simulink library "Vehicule"  (R2018a)
settings: Solver=VariableStepAuto  StartTime=0.0  StopTime=10.0  RelTol=1e-3
values from neighbouring files (symbols this model uses):
  cycleLife = (0:1:500)    [ImportationRoute.m]
  dod = interp1(temperature, deepOfDischarge, temp)    [ImportationRoute.m]
  dod2 = interp1(cyLi, dischargeCapacity, cycleLife)    [ImportationRoute.m]
  temp = (-20:1:40)    [ImportationRoute.m]
libraries: $bdroot x3, simulink x2
settings Model: Creator=thomas.moser  LastModifiedBy=thomas.moser

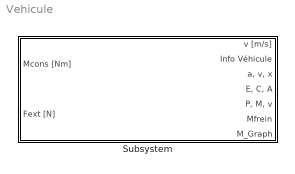
== system Vehicule ==
  Subsystem : Subsystem  mask{m=2250, mp=80, rr=0.33, s=1, cx=0.5, crr=0.015, mlimit=660, alimit=3, Vmin=25/3.6, Vmax=250/3.6, r=9.73, nr=0.9, nm=0.89, Pmax=310380, Mmax=660, nc=0.89, cb=98, soc=100, tempExt=25, nbrCycle=0}
      mask prompts: m "Poids [kg] :"; mp "Poids passagers [kg] :"; rr "Rayon de la roue [m] :"; s "Surface frontale [m^2] :"; cx "Coefficient de trainée [-] :"; crr "Coefficient de résistance aux roulements [-] :"; mlimit "Couple limite [Nm] :"; alimit "Accélération maximum [m/s^2] :"; Vmin "Vitesse minimum pour régénération [km/h] :"; Vmax "Vitesse maximum [km/h]"; r "Rapport de réduction [-] :"; nr "Rendement du réducteur [-] :"; nm "Rendement du moteur [-] :"; Pmax "Puissance maximum [W] :"; Mmax "Couple maximum [Nm] :"; nc "Rendement du convertisseur [-] :"; cb "Capacité de la batterie [kWh] :"; soc "Etat initial de la batterie [%] :"; tempExt "Température extérieure [°C] :"; nbrCycle "Nombre de cycle [-] :"
      mask DialogControl Voiture Prompt: Voiture
      mask DialogControl Transmission Prompt: Bloc moteur
      mask DialogControl Electronique Prompt: Electronique
      mask Display: image('C:\Users\thomas.moser\Documents\GitHub\EV_sim\Photos\Voiture.PNG');

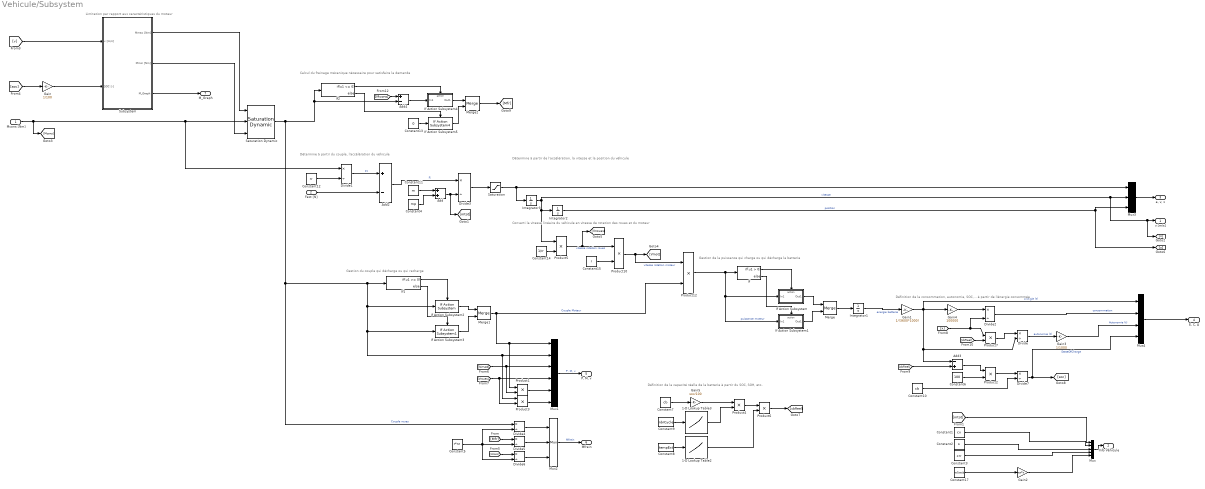
== system Vehicule/Subsystem ==
  note: Définition de la capacité réelle de la batterie à partir du SOC, SOH, etc..
  note: Définition de la consommation, autonomie, SOC,... à partir de l'énergie consommée
  note: Gestion de la puissance qui charge ou qui décharge la batterie
  note: Gestion du couple qui décharge ou qui recharge
  note: Converti la vitesse linéaire du véhicule en vitesse de rotation des roues et du moteur
  note: Détermine à partir de l'accélération, la vitesse et la position du
      | véhicule
  note: Détermine à partir du couple, l'accélération du véhicule
  note: Calcul du freinage mécanique nécessaire pour satisfaire la demande
  note: Limitation par rapport aux caractéristiques du moteur
  Mcons [Nm] : Inport
  Fext [N] : Inport  Port=2
  1-D Lookup Table2 : Lookup_n-D  NumberOfTableDimensions=1  BreakpointsForDimension1=temp  Table=dod  InternalRulePriority=Speed  RndMeth=Simplest  InputSameDT=on
  1-D Lookup Table3 : Lookup_n-D  NumberOfTableDimensions=1  BreakpointsForDimension1=cycleLife  Table=dod2  InternalRulePriority=Speed  RndMeth=Simplest  InputSameDT=on
  Add : Sum
  Add2 : Sum  Inputs=+-
  Add3 : Sum  Inputs=-+
  Add4 : Sum  Inputs=+-
  Constant1 : Constant  Value=cx
  Constant10 : Constant  Value=cb
  Constant11 : Constant  Value=m
  Constant12 : Constant  Value=rr
  Constant13 : Constant  Value=0
  Constant14 : Constant  Value=1/rr
  Constant15 : Constant  Value=r
  Constant17 : Constant  Value=mlimit
  Constant2 : Constant  Value=s
  Constant3 : Constant  Value=crr
  Constant4 : Constant  Value=mp
  Constant5 : Constant  Value=r*nr
  Constant6 : Constant  Value=100
  Constant7 : Constant  Value=cb
  Constant8 : Constant  Value=tempExt
  Constant9 : Constant  Value=nbrCycle
  Divide{,1..7} (8 alike) : Product  Inputs=*/
  Gain : Gain  Gain=1/100
  Gain1 : Gain  Gain=1/(3600*1000)
  Gain2 : Gain  Gain=nr*r
  Gain3 : Gain  Gain=1/1000
  Gain4 : Gain  Gain=100000
  Gain5 : Gain  Gain=soc/100
  If : If
  If Action Subsystem : Subsystem  TreatAsAtomicUnit=on
  If Action Subsystem1 : Subsystem  TreatAsAtomicUnit=on
  If Action Subsystem2 : $bdroot/Subsystem/If Action Subsystem
      link override Constant10: Value=1/nr
      link override Constant18: Value=1/r
  If Action Subsystem3 : $bdroot/Subsystem/If Action Subsystem1
      link override Constant10: Value=1/r
      link override Constant18: Value=nr
  If Action Subsystem4 : Subsystem  TreatAsAtomicUnit=on
  If Action Subsystem5 : $bdroot/Subsystem/If Action Subsystem4
  If1 : If  IfExpression=u1 >= 0
  If2 : If  IfExpression=u1 <= 0
  Integrator1 : Integrator
  Integrator2 : Integrator
  Integrator3 : Integrator
  Merge : Merge
  Merge1 : Merge
  Merge2 : Merge
  Mux : Mux  Inputs=5
  Mux1 : Mux  Inputs=6
  Mux2 : Mux  Inputs=3
  Mux3 : Mux  Inputs=3
  Mux4 : Mux
  Product{1..7,10,12} (9 alike) : Product
  Saturation : Saturate  UpperLimit=alimit  LowerLimit=-alimit
  Saturation Dynamic : simulink/Discontinuities/Saturation Dynamic  OutMin=[]  OutMax=[]  OutDataTypeStr=Inherit: Same as second input  OutDataType=fixdt(1, 16)  OutScaling=2^-10  DoSatur=off
  Subsystem : Subsystem
  v [m/s] : Outport
  Info Véhicule : Outport  Port=2
  "a, v, x" : Outport  Port=3
  "E, C, A" : Outport  Port=4
  "P, M, v" : Outport  Port=5
  Mfrein : Outport  Port=6
  "M_Graph " : Outport  Port=7
  wires:
  Gain3/1 -> Mux4/3  "Autonomie (t)"
  Constant14/1 -> Product5/2
  Product12/1 -> If Action Subsystem/1(In1), If Action Subsystem1/1(In1), If/1  "puissance moteur"
  Integrator3/1 -> Mux3/2, [v], v [m/s]/1, Product5/1, Integrator2/1  "vitesse"
  Constant12/1 -> Divide1/2
  Gain1/1 -> Add3/1, Divide/2, Gain4/1, Mux4/1  "Energie (t)"
  Add2/1 -> Divide3/1  "Fi"
  Mcons [Nm]/1 -> [Mcons], Saturation Dynamic/2, Divide1/1
  Saturation/1 -> Integrator3/1, Mux3/1
  Divide3/1 -> Saturation/1
  Product5/1 -> [Vroues], Product10/1  "vitesse rotation roues"
  Constant15/1 -> Product10/2
  Integrator2/1 -> Mux3/3, [x]  "position"
  Gain4/1 -> Divide2/1
  Divide1/1 -> Add2/1  "Ft"
  Divide2/1 -> Mux4/2  "consommation"
  Divide/1 -> Gain3/1  "autonomie (t)"
  Product10/1 -> [Vmot], Product12/1  "vitesse rotation moteur"
  Fext [N]/1 -> Add2/2
  Constant1/1 -> Mux/2
  Constant2/1 -> Mux/3
  Constant3/1 -> Mux/4
  Mux/1 -> Info Véhicule/1
  Constant4/1 -> Add/2
  Constant11/1 -> Add/1
  Add/1 -> [mtot], Divide3/2
  Integrator1/1 -> Gain1/1  "energie batterie"
  Mux1/1 -> "P, M, v"/1  "P, M, v"
  Saturation Dynamic/1 -> Divide4/1, If Action Subsystem2/1, If Action Subsystem3/1, Product3/1, Mux1/2, If1/1, If2/1, Add4/2  "Couple roues"
  Mux2/1 -> Mfrein/1  "Mfrein"
  Constant5/1 -> Divide6/2, Divide5/2, Divide4/2
  Divide6/1 -> Mux2/3
  Divide5/1 -> Mux2/2
  Divide4/1 -> Mux2/1
  [cbReel] -> Add3/2
  Constant6/1 -> Product2/2
  Add3/1 -> Product2/1
  Product2/1 -> Divide7/1
  Divide7/1 -> [soc], Mux4/4  "StateOfCharge"
  If/1 -> If Action Subsystem/Action
  If/2 -> If Action Subsystem1/Action
  If Action Subsystem/1(Out1) -> Merge/1
  If Action Subsystem1/1(Out1) -> Merge/2
  Merge/1 -> Integrator1/1
  Merge1/1 -> Product1/1, Mux1/1, Product12/2  "Couple Moteur"
  If Action Subsystem3/1 -> Merge1/2
  If Action Subsystem2/1 -> Merge1/1
  If1/2 -> If Action Subsystem3/Action
  If1/1 -> If Action Subsystem2/Action
  Mux3/1 -> "a, v, x"/1
  Mux4/1 -> "E, C, A"/1
  [Mfr] -> Divide5/1
  [mtot] -> Mux/1
  [Mcons] -> Divide6/1
  [Vmot] -> Product1/2, Mux1/3
  [Vroues] -> Product3/2, Mux1/4
  Product3/1 -> Mux1/6
  Product1/1 -> Mux1/5
  [x] -> Product7/1, Divide2/2
  Constant7/1 -> Gain5/1
  Constant8/1 -> 1-D Lookup Table2/1
  Constant9/1 -> 1-D Lookup Table3/1
  Gain5/1 -> Product4/1
  Product4/1 -> Product6/1
  1-D Lookup Table2/1 -> Product6/2
  Product6/1 -> [cbReel]
  Product7/1 -> Divide/1
  [cbReel] -> Product7/2
  1-D Lookup Table3/1 -> Product4/2
  Constant10/1 -> Divide7/2
  [v] -> Subsystem/1(v [m/s])
  Subsystem/2(Mmin [Nm]) -> Saturation Dynamic/3
  If2/1 -> If Action Subsystem4/Action
  [Mcons] -> Add4/1
  Add4/1 -> If Action Subsystem4/1(In1)
  If Action Subsystem4/1(Out1) -> Merge2/1
  If2/2 -> If Action Subsystem5/Action
  Constant13/1 -> If Action Subsystem5/1
  If Action Subsystem5/1 -> Merge2/2
  Merge2/1 -> [Mfr]
  [soc] -> Gain/1
  Gain/1 -> Subsystem/2(SOC [-])
  Constant17/1 -> Gain2/1
  Subsystem/1(Mmax [Nm]) -> Saturation Dynamic/1
  Subsystem/3(M_Graph) -> "M_Graph "/1
  Gain2/1 -> Mux/5

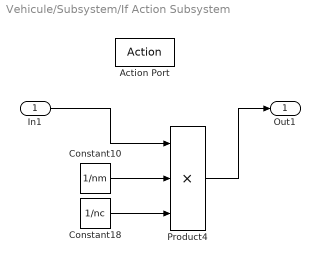
== system Vehicule/Subsystem/If Action Subsystem ==
  In1 : Inport
  Action Port : ActionPort  ActionType=then
  Constant10 : Constant  Value=1/nm
  Constant18 : Constant  Value=1/nc
  Product4 : Product  Inputs=3
  Out1 : Outport
  wires:
  Constant18/1 -> Product4/3
  Constant10/1 -> Product4/2
  In1/1 -> Product4/1
  Product4/1 -> Out1/1

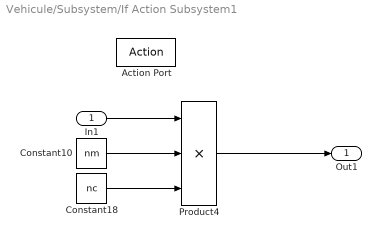
== system Vehicule/Subsystem/If Action Subsystem1 ==
  In1 : Inport
  Action Port : ActionPort  ActionType=else
  Constant10 : Constant  Value=nm
  Constant18 : Constant  Value=nc
  Product4 : Product  Inputs=3
  Out1 : Outport
  wires:
  Constant18/1 -> Product4/3
  Constant10/1 -> Product4/2
  In1/1 -> Product4/1
  Product4/1 -> Out1/1

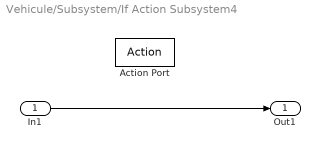
== system Vehicule/Subsystem/If Action Subsystem4 ==
  In1 : Inport
  Action Port : ActionPort  ActionType=then
  Out1 : Outport
  wires:
  In1/1 -> Out1/1

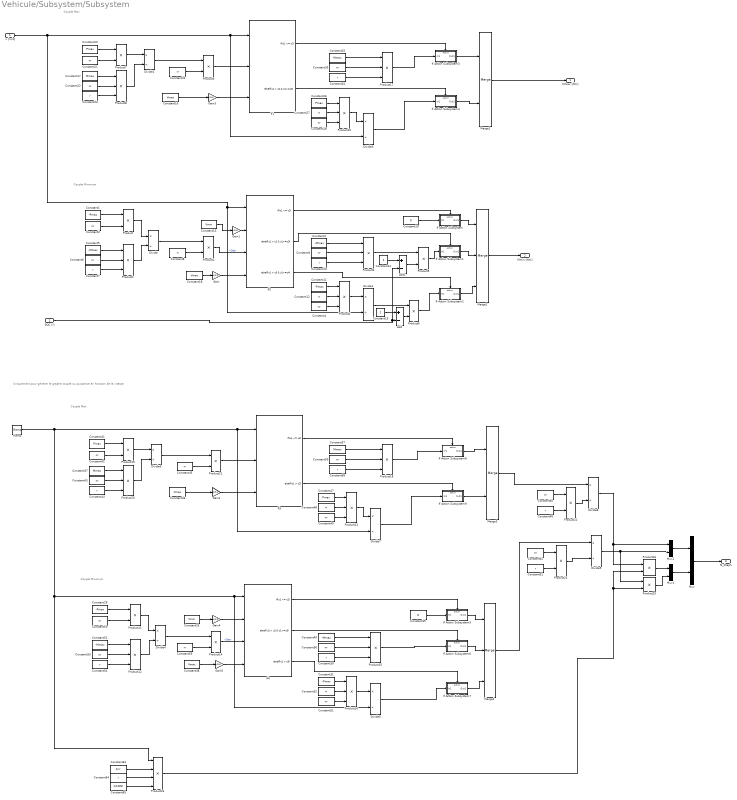
== system Vehicule/Subsystem/Subsystem ==
  note: Uniquement pour générer le graphe couple ou puissance en fonction de la vitesse
  note: Couple Minimum
  note: Couple Max
  note: Couple Minimum
  note: Couple Max
  v [m/s] : Inport
  SOC [-] : Inport  Port=2
  Add : Sum  Inputs=+-
  Add1 : Sum  Inputs=+-
  Constant{1,11,29,31} (4 alike) : Constant  Value=-Pmax
  Constant{7,10,23,30,34,44,46,54,58,61,64} (11 alike) : Constant  Value=r
  Constant{8,12,24,27,32,45,48,55} (8 alike) : Constant  Value=rr
  Constant13 : Constant  Value=Vmin
  Constant14 : Constant
  Constant15 : Constant
  Constant{16,18,36,38} (4 alike) : Constant  Value=Vmax
  Constant{17,25,37,57} (4 alike) : Constant  Value=Mmax
  Constant19 : Constant  Value=0
  Constant{2,5,40,52} (4 alike) : Constant  Value=-Mmax
  Constant{20,26,41,47} (4 alike) : Constant  Value=Pmax
  Constant{3..4,6,9,21..22,28,35,42..43,49..51,53,56,59..60,62} (18 alike) : Constant  Value=nr
  Constant33 : Constant  Value=Vmin
  Constant39 : Constant  Value=0
  Constant63 : Constant  Value=1/rr
  Constant65 : Constant  Value=1/1000
  Divide{,1..9} (10 alike) : Product  Inputs=*/
  Gain{,1..5} (6 alike) : Gain  Gain=1/3.6
  If Action Subsystem : Subsystem  TreatAsAtomicUnit=on
  If Action Subsystem1 : Subsystem  TreatAsAtomicUnit=on
  If Action Subsystem2 : Subsystem  TreatAsAtomicUnit=on
  If Action Subsystem3 : Subsystem  TreatAsAtomicUnit=on
  If Action Subsystem4 : Subsystem  TreatAsAtomicUnit=on
  If Action Subsystem5 : Subsystem  TreatAsAtomicUnit=on
  If Action Subsystem6 : Subsystem  TreatAsAtomicUnit=on
  If Action Subsystem7 : Subsystem  TreatAsAtomicUnit=on
  If Action Subsystem8 : Subsystem  TreatAsAtomicUnit=on
  If Action Subsystem9 : Subsystem  TreatAsAtomicUnit=on
  If1 : If  NumInputs=3  IfExpression=u1 <= u2  ElseIfExpressions=u1 > u2 & u1<=u3  ShowElse=off
  If2 : If  NumInputs=4  IfExpression=u1 <= u2  ElseIfExpressions=u1 > u2 & u1<=u3, u1 > u3 & u1<=u4  ShowElse=off
  If3 : If  NumInputs=3  IfExpression=u1 <= u2  ElseIfExpressions=u1 > u2  ShowElse=off
  If4 : If  NumInputs=4  IfExpression=u1 <= u2  ElseIfExpressions=u1 > u2 & u1<=u3, u1 > u3  ShowElse=off
  Merge1 : Merge
  Merge2 : Merge  Inputs=3
  Merge3 : Merge
  Merge4 : Merge  Inputs=3
  Mux : Mux  Inputs=2
  Mux1 : Mux  Inputs=2
  Mux2 : Mux  Inputs=2
  Product{,2,5..7,9,11,14,19,21..23,25..26} (14 alike) : Product
  Product{1,3..4,8,10,12..13,15..18,20} (12 alike) : Product  Inputs=3
  Product24 : Product  Inputs=4
  Ramp : simulink/Sources/Ramp  slope=1  start=0  InitialOutput=0
  Mmax [Nm] : Outport
  Mmin [Nm] : Outport  Port=2
  M_Graph : Outport  Port=3
  wires:
  If2/1 -> If Action Subsystem/Action
  Product2/1 -> If2/3  "VDecr"
  Constant4/1 -> Product4/3
  Constant2/1 -> Product3/1
  Product1/1 -> Divide/2
  Constant18/1 -> Gain/1
  Product/1 -> Divide/1
  Constant7/1 -> Product1/3
  Add1/1 -> Product5/2
  Constant1/1 -> Product/1
  v [m/s]/1 -> Divide1/2, If2/1, Divide3/2, If1/1
  If2/2 -> If Action Subsystem1/Action
  Divide1/1 -> Product6/1
  Constant3/1 -> Product/2
  Divide/1 -> Product2/1
  Add/1 -> Product6/2
  Constant5/1 -> Product1/1
  Constant6/1 -> Product1/2
  Constant11/1 -> Product4/1
  Constant19/1 -> If Action Subsystem/1(In1)
  Constant9/1 -> Product3/2
  If Action Subsystem/1(Out1) -> Merge2/1
  If Action Subsystem2/1(Out1) -> Merge2/3
  SOC [-]/1 -> Add1/2, Add/2
  Constant13/1 -> Gain1/1
  Product6/1 -> If Action Subsystem2/1(In1)
  Constant14/1 -> Add1/1
  Product5/1 -> If Action Subsystem1/1(In1)
  If Action Subsystem1/1(Out1) -> Merge2/2
  Merge2/1 -> Mmin [Nm]/1
  If2/3 -> If Action Subsystem2/Action
  Product4/1 -> Divide1/1
  Product3/1 -> Product5/1
  Constant12/1 -> Product4/2
  Constant10/1 -> Product3/3
  Constant8/1 -> Product2/2
  Constant15/1 -> Add/1
  Constant16/1 -> Gain3/1
  Constant20/1 -> Product7/1
  Constant21/1 -> Product7/2
  Constant17/1 -> Product8/1
  Constant22/1 -> Product8/2
  Constant23/1 -> Product8/3
  Product8/1 -> Divide2/2
  Product7/1 -> Divide2/1
  Divide2/1 -> Product9/1
  Constant24/1 -> Product9/2
  Product9/1 -> If1/2
  If1/1 -> If Action Subsystem3/Action
  Constant25/1 -> Product17/1
  If Action Subsystem3/1(Out1) -> Merge1/1
  If1/2 -> If Action Subsystem4/Action
  Constant26/1 -> Product10/1
  Constant27/1 -> Product10/2
  Constant28/1 -> Product10/3
  Product10/1 -> Divide3/1
  Divide3/1 -> If Action Subsystem4/1(In1)
  If Action Subsystem4/1(Out1) -> Merge1/2
  Merge1/1 -> Mmax [Nm]/1
  Divide7/1 -> If Action Subsystem9/1(In1)
  If Action Subsystem9/1(Out1) -> Merge3/2
  Product19/1 -> Divide6/1
  If Action Subsystem5/1(Out1) -> Merge4/1
  Constant54/1 -> Product12/3
  Constant56/1 -> Product15/2
  Constant32/1 -> Product16/2
  Product16/1 -> Divide5/1
  If Action Subsystem6/1(Out1) -> Merge4/2
  Constant39/1 -> If Action Subsystem5/1(In1)
  Constant31/1 -> Product16/1
  Constant30/1 -> Product15/3
  Constant55/1 -> Product14/2
  If4/3 -> If Action Subsystem7/Action
  Constant37/1 -> Product20/1
  Constant43/1 -> Product20/2
  Divide6/1 -> Product21/1
  Constant38/1 -> Gain5/1
  Divide4/1 -> Product14/1
  If4/2 -> If Action Subsystem6/Action
  Constant50/1 -> Product11/2
  If4/1 -> If Action Subsystem5/Action
  Divide5/1 -> If Action Subsystem7/1(In1)
  Product11/1 -> Divide4/1
  Constant36/1 -> Gain2/1
  Product13/1 -> Divide7/1
  Ramp/1 -> Product24/1, Divide5/2, If4/1, Divide7/2, If3/1
  Constant29/1 -> Product11/1
  Product12/1 -> Divide4/2
  Product14/1 -> If4/3  "VDecr"
  Constant51/1 -> Product16/3
  If Action Subsystem7/1(Out1) -> Merge4/3
  Constant42/1 -> Product19/2
  Product20/1 -> Divide6/2
  Constant53/1 -> Product12/2
  Constant33/1 -> Gain4/1
  Product21/1 -> If3/2
  Constant52/1 -> Product12/1
  If3/1 -> If Action Subsystem8/Action
  Constant40/1 -> Product15/1
  Constant47/1 -> Product13/1
  Constant49/1 -> Product13/3
  Constant48/1 -> Product13/2
  Constant41/1 -> Product19/1
  If Action Subsystem8/1(Out1) -> Merge3/1
  Constant44/1 -> Product20/3
  Merge3/1 -> Divide8/1
  Constant45/1 -> Product21/2
  If3/2 -> If Action Subsystem9/Action
  Product15/1 -> If Action Subsystem6/1(In1)
  Mux/1 -> M_Graph/1
  Constant35/1 -> Product17/2
  Constant34/1 -> Product17/3
  Product17/1 -> If Action Subsystem3/1(In1)
  Constant59/1 -> Product18/2
  Constant57/1 -> Product18/1
  Constant58/1 -> Product18/3
  Product18/1 -> If Action Subsystem8/1(In1)
  Gain/1 -> If2/4
  Gain1/1 -> If2/2
  Gain2/1 -> If3/3
  Gain3/1 -> If1/3
  Gain4/1 -> If4/2
  Gain5/1 -> If4/4
  Constant60/1 -> Product22/1
  Constant46/1 -> Product22/2
  Product22/1 -> Divide8/2
  Divide8/1 -> Mux2/1, Product26/1
  Constant61/1 -> Product23/2
  Product23/1 -> Divide9/2
  Constant62/1 -> Product23/1
  Divide9/1 -> Product25/1, Mux2/2
  Merge4/1 -> Divide9/1
  Constant63/1 -> Product24/2
  Constant64/1 -> Product24/3
  Product24/1 -> Product26/2, Product25/2
  Product25/1 -> Mux1/2
  Product26/1 -> Mux1/1
  Constant65/1 -> Product24/4
  Mux2/1 -> Mux/1
  Mux1/1 -> Mux/2

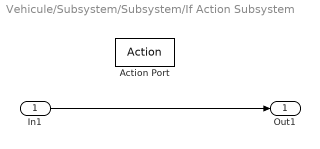
== system Vehicule/Subsystem/Subsystem/If Action Subsystem ==
  In1 : Inport
  Action Port : ActionPort
  Out1 : Outport
  wires:
  In1/1 -> Out1/1

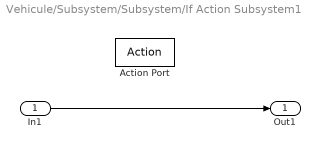
== system Vehicule/Subsystem/Subsystem/If Action Subsystem1 ==
  In1 : Inport
  Action Port : ActionPort
  Out1 : Outport
  wires:
  In1/1 -> Out1/1

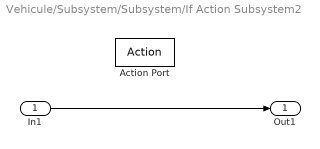
== system Vehicule/Subsystem/Subsystem/If Action Subsystem2 ==
  In1 : Inport
  Action Port : ActionPort
  Out1 : Outport
  wires:
  In1/1 -> Out1/1

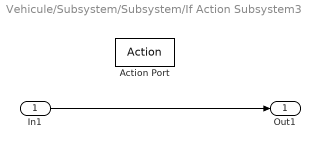
== system Vehicule/Subsystem/Subsystem/If Action Subsystem3 ==
  In1 : Inport
  Action Port : ActionPort
  Out1 : Outport
  wires:
  In1/1 -> Out1/1

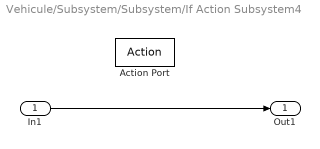
== system Vehicule/Subsystem/Subsystem/If Action Subsystem4 ==
  In1 : Inport
  Action Port : ActionPort
  Out1 : Outport
  wires:
  In1/1 -> Out1/1

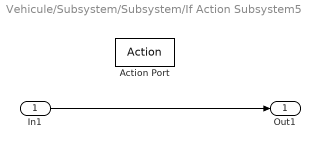
== system Vehicule/Subsystem/Subsystem/If Action Subsystem5 ==
  In1 : Inport
  Action Port : ActionPort
  Out1 : Outport
  wires:
  In1/1 -> Out1/1

== system Vehicule/Subsystem/Subsystem/If Action Subsystem6 ==
  In1 : Inport
  Action Port : ActionPort
  Out1 : Outport
  wires:
  In1/1 -> Out1/1

== system Vehicule/Subsystem/Subsystem/If Action Subsystem7 ==
  In1 : Inport
  Action Port : ActionPort
  Out1 : Outport
  wires:
  In1/1 -> Out1/1

== system Vehicule/Subsystem/Subsystem/If Action Subsystem8 ==
  In1 : Inport
  Action Port : ActionPort
  Out1 : Outport
  wires:
  In1/1 -> Out1/1

== system Vehicule/Subsystem/Subsystem/If Action Subsystem9 ==
  In1 : Inport
  Action Port : ActionPort
  Out1 : Outport
  wires:
  In1/1 -> Out1/1
